simulink model "casper_sim_phase0"  (R2025b)
settings: Solver=FixedStepDiscrete  StartTime=0  StopTime=5  FixedStep=1e-3  RelTol=1e-3
undefined symbols (not defined in the file or in its folder): Estimator
libraries: imu_block_visual x2, baro_block_visual x1, gps_block_visual x1, mag_block_visual x1
settings Model: Creator=Ashwin  LastModifiedBy=Ashwin
settings DebuggingCC: InheritedTsInSrcMsg=none

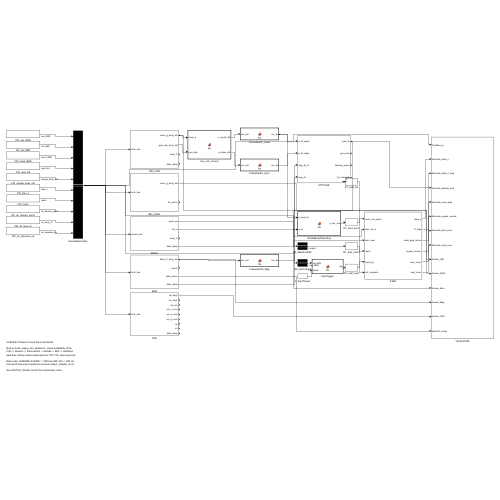
[thumbnail: Simulink's stored preview of the top-level diagram]
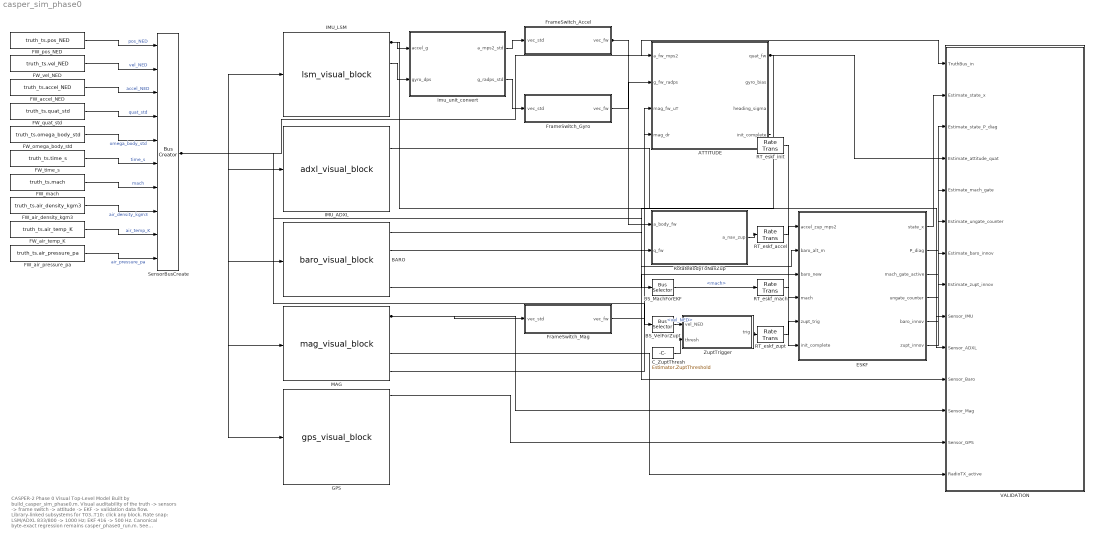
== system casper_sim_phase0 ==
  note: CASPER-2 Phase 0 Visual Top-Level Model
      |
      | Built by build_casper_sim_phase0.m. Visual auditability of the
      | truth -> sensors -> frame switch -> attitude -> EKF -> validation
      | data flow. Library-linked subsystems for T03..T10; click any block.
      |
      | Rate snap: LSM/ADXL 833/800 -> 1000 Hz; EKF 416 -> 500 Hz.
      | Canonical byte-exact regression remains casper_phase0_run.m.
      |
      | See STATUS_VISUAL.md for the construction notes.
  ATTITUDE : Subsystem
  BARO : baro_block_visual/baro_visual_block  SystemSampleTime=-1  VariantActivationTime=update diagram  EmptyChoice=off  PassThrough=off  PassThroughVariantControl=(default)  EmptyChoiceVariantControl=(default)  AllowFlexibleInterface=on  Latency=0  AutoFrameSizeCalculation=off
  BS_MachForEKF : BusSelector  OutputSignals=mach
  BS_VelForZupt : BusSelector  OutputSignals=vel_NED
  C_ZuptThresh : Constant  Value=Estimator.ZuptThreshold  SampleTime=-1
  ESKF : Subsystem
  FW_accel_NED : FromWorkspace  VariableName=truth_ts.accel_NED  SampleTime=-1  ZeroCross=off  OutputAfterFinalValue=Holding final value
  FW_air_density_kgm3 : FromWorkspace  VariableName=truth_ts.air_density_kgm3  SampleTime=-1  ZeroCross=off  OutputAfterFinalValue=Holding final value
  FW_air_pressure_pa : FromWorkspace  VariableName=truth_ts.air_pressure_pa  SampleTime=-1  ZeroCross=off  OutputAfterFinalValue=Holding final value
  FW_air_temp_K : FromWorkspace  VariableName=truth_ts.air_temp_K  SampleTime=-1  ZeroCross=off  OutputAfterFinalValue=Holding final value
  FW_mach : FromWorkspace  VariableName=truth_ts.mach  SampleTime=-1  ZeroCross=off  OutputAfterFinalValue=Holding final value
  FW_omega_body_std : FromWorkspace  VariableName=truth_ts.omega_body_std  SampleTime=-1  ZeroCross=off  OutputAfterFinalValue=Holding final value
  FW_pos_NED : FromWorkspace  VariableName=truth_ts.pos_NED  SampleTime=-1  ZeroCross=off  OutputAfterFinalValue=Holding final value
  FW_quat_std : FromWorkspace  VariableName=truth_ts.quat_std  SampleTime=-1  ZeroCross=off  OutputAfterFinalValue=Holding final value
  FW_time_s : FromWorkspace  VariableName=truth_ts.time_s  SampleTime=-1  ZeroCross=off  OutputAfterFinalValue=Holding final value
  FW_vel_NED : FromWorkspace  VariableName=truth_ts.vel_NED  SampleTime=-1  ZeroCross=off  OutputAfterFinalValue=Holding final value
  FrameSwitch_Accel : MATLAB Function  TreatAsAtomicUnit=on
  FrameSwitch_Gyro : MATLAB Function  TreatAsAtomicUnit=on
  FrameSwitch_Mag : MATLAB Function  TreatAsAtomicUnit=on
  GPS : gps_block_visual/gps_visual_block  SystemSampleTime=-1  VariantActivationTime=update diagram  EmptyChoice=off  PassThrough=off  PassThroughVariantControl=(default)  EmptyChoiceVariantControl=(default)  AllowFlexibleInterface=on  Latency=0  AutoFrameSizeCalculation=off
  IMU_ADXL : imu_block_visual/adxl_visual_block  SystemSampleTime=-1  VariantActivationTime=update diagram  EmptyChoice=off  PassThrough=off  PassThroughVariantControl=(default)  EmptyChoiceVariantControl=(default)  AllowFlexibleInterface=on  Latency=0  AutoFrameSizeCalculation=off
  IMU_LSM : imu_block_visual/lsm_visual_block  SystemSampleTime=-1  VariantActivationTime=update diagram  EmptyChoice=off  PassThrough=off  PassThroughVariantControl=(default)  EmptyChoiceVariantControl=(default)  AllowFlexibleInterface=on  Latency=0  AutoFrameSizeCalculation=off
  MAG : mag_block_visual/mag_visual_block  SystemSampleTime=-1  VariantActivationTime=update diagram  EmptyChoice=off  PassThrough=off  PassThroughVariantControl=(default)  EmptyChoiceVariantControl=(default)  AllowFlexibleInterface=on  Latency=0  AutoFrameSizeCalculation=off
  RT_eskf_accel : RateTransition  OutPortSampleTime=2e-3
  RT_eskf_init : RateTransition  OutPortSampleTime=2e-3
  RT_eskf_mach : RateTransition  OutPortSampleTime=2e-3
  RT_eskf_zupt : RateTransition  OutPortSampleTime=2e-3
  RotateBodyToNavZup : MATLAB Function  TreatAsAtomicUnit=on
  SensorBusCreate : BusCreator  Inputs=10  OutDataTypeStr=Bus: SensorInputBus  NonVirtualBus=on
  VALIDATION : Subsystem
  ZuptTrigger : MATLAB Function  TreatAsAtomicUnit=on
  imu_unit_convert : MATLAB Function  TreatAsAtomicUnit=on
  wires:
  FW_pos_NED/1 -> SensorBusCreate/1  "pos_NED"
  FW_vel_NED/1 -> SensorBusCreate/2  "vel_NED"
  FW_accel_NED/1 -> SensorBusCreate/3  "accel_NED"
  FW_quat_std/1 -> SensorBusCreate/4  "quat_std"
  FW_omega_body_std/1 -> SensorBusCreate/5  "omega_body_std"
  FW_time_s/1 -> SensorBusCreate/6  "time_s"
  FW_mach/1 -> SensorBusCreate/7  "mach"
  FW_air_density_kgm3/1 -> SensorBusCreate/8  "air_density_kgm3"
  FW_air_temp_K/1 -> SensorBusCreate/9  "air_temp_K"
  FW_air_pressure_pa/1 -> SensorBusCreate/10  "air_pressure_pa"
  SensorBusCreate/1 -> IMU_LSM/1, IMU_ADXL/1, BARO/1, MAG/1, GPS/1, BS_MachForEKF/1, BS_VelForZupt/1, VALIDATION/1(TruthBus_in)
  IMU_LSM/1 -> imu_unit_convert/1(accel_g), VALIDATION/9(Sensor_IMU)
  IMU_LSM/2 -> imu_unit_convert/2(gyro_dps)
  imu_unit_convert/1(a_mps2_std) -> FrameSwitch_Accel/1(vec_std)
  imu_unit_convert/2(g_radps_std) -> FrameSwitch_Gyro/1(vec_std)
  MAG/1 -> FrameSwitch_Mag/1(vec_std), VALIDATION/12(Sensor_Mag)
  FrameSwitch_Accel/1(vec_fw) -> ATTITUDE/1(a_fw_mps2), RotateBodyToNavZup/1(a_body_fw)
  FrameSwitch_Gyro/1(vec_fw) -> ATTITUDE/2(g_fw_radps)
  FrameSwitch_Mag/1(vec_fw) -> ATTITUDE/3(mag_fw_uT)
  MAG/4 -> ATTITUDE/4(mag_dr)
  ATTITUDE/1(quat_fw) -> RotateBodyToNavZup/2(q_fw), VALIDATION/4(Estimate_attitude_quat)
  RotateBodyToNavZup/1(a_nav_zup) -> RT_eskf_accel/1
  BS_MachForEKF/1 -> RT_eskf_mach/1  "<mach>"
  BS_VelForZupt/1 -> ZuptTrigger/1(vel_NED)  "<vel_NED>"
  C_ZuptThresh/1 -> ZuptTrigger/2(thresh)
  ZuptTrigger/1(trig) -> RT_eskf_zupt/1
  ATTITUDE/4(init_complete) -> RT_eskf_init/1
  RT_eskf_accel/1 -> ESKF/1(accel_zup_mps2)
  BARO/2 -> ESKF/2(baro_alt_m)
  BARO/4 -> ESKF/3(baro_new)
  RT_eskf_mach/1 -> ESKF/4(mach)
  RT_eskf_zupt/1 -> ESKF/5(zupt_trig)
  RT_eskf_init/1 -> ESKF/6(init_complete)
  ESKF/1(state_x) -> VALIDATION/2(Estimate_state_x)
  ESKF/2(P_diag) -> VALIDATION/3(Estimate_state_P_diag)
  ESKF/3(mach_gate_active) -> VALIDATION/5(Estimate_mach_gate)
  ESKF/4(ungate_counter) -> VALIDATION/6(Estimate_ungate_counter)
  ESKF/5(baro_innov) -> VALIDATION/7(Estimate_baro_innov)
  ESKF/6(zupt_innov) -> VALIDATION/8(Estimate_zupt_innov)
  IMU_ADXL/1 -> VALIDATION/10(Sensor_ADXL)
  BARO/1 -> VALIDATION/11(Sensor_Baro)
  GPS/1 -> VALIDATION/13(Sensor_GPS)
  MAG/3 -> VALIDATION/14(RadioTX_active)

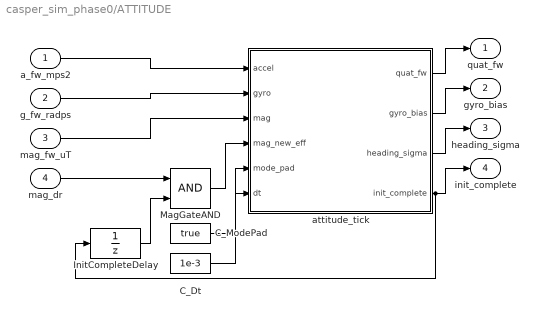
== system casper_sim_phase0/ATTITUDE ==
  a_fw_mps2 : Inport
  g_fw_radps : Inport  Port=2
  mag_fw_uT : Inport  Port=3
  mag_dr : Inport  Port=4
  C_Dt : Constant  Value=1e-3  SampleTime=-1
  C_ModePad : Constant  Value=true  OutDataTypeStr=boolean  SampleTime=-1
  InitCompleteDelay : UnitDelay  SampleTime=-1  HasFrameUpgradeWarning=on
  MagGateAND : Logic  AllPortsSameDT=off  OutDataTypeStr=boolean
  attitude_tick : MATLAB Function  TreatAsAtomicUnit=on
  quat_fw : Outport
  gyro_bias : Outport  Port=2
  heading_sigma : Outport  Port=3
  init_complete : Outport  Port=4
  wires:
  mag_dr/1 -> MagGateAND/1
  InitCompleteDelay/1 -> MagGateAND/2
  a_fw_mps2/1 -> attitude_tick/1(accel)
  g_fw_radps/1 -> attitude_tick/2(gyro)
  mag_fw_uT/1 -> attitude_tick/3(mag)
  MagGateAND/1 -> attitude_tick/4(mag_new_eff)
  C_ModePad/1 -> attitude_tick/5(mode_pad)
  C_Dt/1 -> attitude_tick/6(dt)
  attitude_tick/4(init_complete) -> InitCompleteDelay/1, init_complete/1
  attitude_tick/1(quat_fw) -> quat_fw/1
  attitude_tick/2(gyro_bias) -> gyro_bias/1
  attitude_tick/3(heading_sigma) -> heading_sigma/1

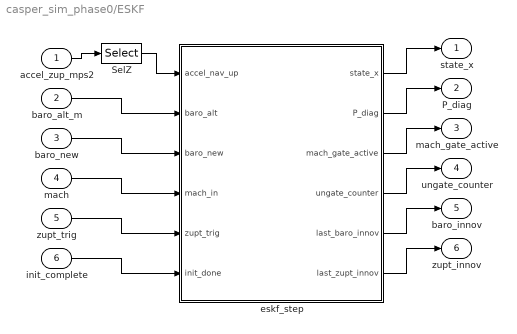
== system casper_sim_phase0/ESKF ==
  accel_zup_mps2 : Inport
  baro_alt_m : Inport  Port=2
  baro_new : Inport  Port=3
  mach : Inport  Port=4
  zupt_trig : Inport  Port=5
  init_complete : Inport  Port=6
  SelZ : Selector  InputPortWidth=3  IndexOptions=Index vector (dialog)  Indices=3  OutputSizes=1
  eskf_step : MATLAB Function  TreatAsAtomicUnit=on
  state_x : Outport
  P_diag : Outport  Port=2
  mach_gate_active : Outport  Port=3
  ungate_counter : Outport  Port=4
  baro_innov : Outport  Port=5
  zupt_innov : Outport  Port=6
  wires:
  accel_zup_mps2/1 -> SelZ/1
  SelZ/1 -> eskf_step/1(accel_nav_up)
  baro_alt_m/1 -> eskf_step/2(baro_alt)
  baro_new/1 -> eskf_step/3(baro_new)
  mach/1 -> eskf_step/4(mach_in)
  zupt_trig/1 -> eskf_step/5(zupt_trig)
  init_complete/1 -> eskf_step/6(init_done)
  eskf_step/1(state_x) -> state_x/1
  eskf_step/2(P_diag) -> P_diag/1
  eskf_step/3(mach_gate_active) -> mach_gate_active/1
  eskf_step/4(ungate_counter) -> ungate_counter/1
  eskf_step/5(last_baro_innov) -> baro_innov/1
  eskf_step/6(last_zupt_innov) -> zupt_innov/1

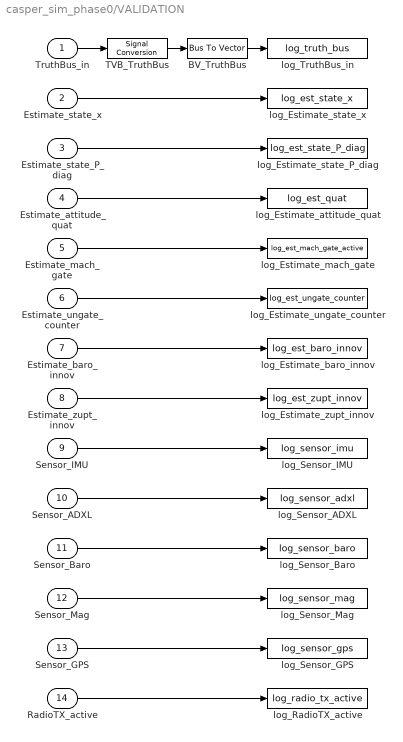
== system casper_sim_phase0/VALIDATION ==
  TruthBus_in : Inport
  Estimate_state_x : Inport  Port=2
  Estimate_state_P_diag : Inport  Port=3
  Estimate_attitude_quat : Inport  Port=4
  Estimate_mach_gate : Inport  Port=5
  Estimate_ungate_counter : Inport  Port=6
  Estimate_baro_innov : Inport  Port=7
  Estimate_zupt_innov : Inport  Port=8
  Sensor_IMU : Inport  Port=9
  Sensor_ADXL : Inport  Port=10
  Sensor_Baro : Inport  Port=11
  Sensor_Mag : Inport  Port=12
  Sensor_GPS : Inport  Port=13
  RadioTX_active : Inport  Port=14
  BV_TruthBus : BusToVector
  TVB_TruthBus : SignalConversion  ConversionOutput=Virtual bus  OverrideOpt=off
  log_Estimate_attitude_quat : ToWorkspace  VariableName=log_est_quat  SaveFormat=Structure With Time  SampleTime=-1
  log_Estimate_baro_innov : ToWorkspace  VariableName=log_est_baro_innov  SaveFormat=Structure With Time  SampleTime=-1
  log_Estimate_mach_gate : ToWorkspace  VariableName=log_est_mach_gate_active  SaveFormat=Structure With Time  SampleTime=-1
  log_Estimate_state_P_diag : ToWorkspace  VariableName=log_est_state_P_diag  SaveFormat=Structure With Time  SampleTime=-1
  log_Estimate_state_x : ToWorkspace  VariableName=log_est_state_x  SaveFormat=Structure With Time  SampleTime=-1
  log_Estimate_ungate_counter : ToWorkspace  VariableName=log_est_ungate_counter  SaveFormat=Structure With Time  SampleTime=-1
  log_Estimate_zupt_innov : ToWorkspace  VariableName=log_est_zupt_innov  SaveFormat=Structure With Time  SampleTime=-1
  log_RadioTX_active : ToWorkspace  VariableName=log_radio_tx_active  SaveFormat=Structure With Time  SampleTime=-1
  log_Sensor_ADXL : ToWorkspace  VariableName=log_sensor_adxl  SaveFormat=Structure With Time  SampleTime=-1
  log_Sensor_Baro : ToWorkspace  VariableName=log_sensor_baro  SaveFormat=Structure With Time  SampleTime=-1
  log_Sensor_GPS : ToWorkspace  VariableName=log_sensor_gps  SaveFormat=Structure With Time  SampleTime=-1
  log_Sensor_IMU : ToWorkspace  VariableName=log_sensor_imu  SaveFormat=Structure With Time  SampleTime=-1
  log_Sensor_Mag : ToWorkspace  VariableName=log_sensor_mag  SaveFormat=Structure With Time  SampleTime=-1
  log_TruthBus_in : ToWorkspace  VariableName=log_truth_bus  SaveFormat=Structure With Time  SampleTime=-1
  wires:
  TruthBus_in/1 -> TVB_TruthBus/1
  TVB_TruthBus/1 -> BV_TruthBus/1
  BV_TruthBus/1 -> log_TruthBus_in/1
  Estimate_state_x/1 -> log_Estimate_state_x/1
  Estimate_state_P_diag/1 -> log_Estimate_state_P_diag/1
  Estimate_attitude_quat/1 -> log_Estimate_attitude_quat/1
  Estimate_mach_gate/1 -> log_Estimate_mach_gate/1
  Estimate_ungate_counter/1 -> log_Estimate_ungate_counter/1
  Estimate_baro_innov/1 -> log_Estimate_baro_innov/1
  Estimate_zupt_innov/1 -> log_Estimate_zupt_innov/1
  Sensor_IMU/1 -> log_Sensor_IMU/1
  Sensor_ADXL/1 -> log_Sensor_ADXL/1
  Sensor_Baro/1 -> log_Sensor_Baro/1
  Sensor_Mag/1 -> log_Sensor_Mag/1
  Sensor_GPS/1 -> log_Sensor_GPS/1
  RadioTX_active/1 -> log_RadioTX_active/1

== matlab function casper_sim_phase0/FrameSwitch_Accel ==
  data: vec_std input; vec_fw output
function vec_fw = fcn(vec_std)
%#codegen
v = double(vec_std(:));
vec_fw = [ v(2); v(1); -v(3) ];
end

== matlab function casper_sim_phase0/imu_unit_convert ==
  data: accel_g input; a_mps2_std output; gyro_dps input; g_radps_std output
function [a_mps2_std, g_radps_std] = fcn(accel_g, gyro_dps)
%#codegen
a_mps2_std  = double(accel_g(:)) * 9.80665;
g_radps_std = double(gyro_dps(:)) * (pi/180);
end

== matlab function casper_sim_phase0/FrameSwitch_Gyro ==
  data: vec_std input; vec_fw output
function vec_fw = fcn(vec_std)
%#codegen
v = double(vec_std(:));
vec_fw = [ v(2); v(1); -v(3) ];
end

== matlab function casper_sim_phase0/FrameSwitch_Mag ==
  data: vec_std input; vec_fw output
function vec_fw = fcn(vec_std)
%#codegen
v = double(vec_std(:));
vec_fw = [ v(2); v(1); -v(3) ];
end

== matlab function casper_sim_phase0/ATTITUDE/attitude_tick ==
  data: accel input; quat_fw output; gyro input; mag input; mag_new_eff input; mode_pad input; dt input; gyro_bias output; heading_sigma output; init_complete output
function [quat_fw, gyro_bias, heading_sigma, init_complete] = fcn(accel, gyro, mag, mag_new_eff, mode_pad, dt)
%#codegen
coder.extrinsic('attitude_step_helper');
% Preallocate outputs so chart parser can infer types.
quat_fw       = [1;0;0;0];
gyro_bias     = zeros(3,1);
heading_sigma = double(0);
init_complete = false;
[quat_fw, gyro_bias, heading_sigma, init_complete] = attitude_step_helper(double(accel), double(gyro), double(mag), logical(mag_new_eff), logical(mode_pad), double(dt));
end

== matlab function casper_sim_phase0/ESKF/eskf_step ==
  data: accel_nav_up input; state_x output; baro_alt input; baro_new input; mach_in input; zupt_trig input; init_done input; P_diag output; mach_gate_active output; ungate_counter output; last_baro_innov output; last_zupt_innov output
function [state_x, P_diag, mach_gate_active, ungate_counter, last_baro_innov, last_zupt_innov] = fcn(accel_nav_up, baro_alt, baro_new, mach_in, zupt_trig, init_done)
%#codegen
coder.extrinsic('eskf_step_helper');
% All outputs preallocated to fixed sizes so the chart parser can
% statically infer types even with extrinsic call.
state_x = zeros(4,1);
P_diag  = zeros(4,1);
mach_gate_active = double(0);
ungate_counter   = double(0);
last_baro_innov  = double(0);
last_zupt_innov  = double(0);
[state_x, P_diag, mach_gate_active, ungate_counter, last_baro_innov, last_zupt_innov] = eskf_step_helper(double(accel_nav_up), double(baro_alt), logical(baro_new), double(mach_in), logical(zupt_trig), logical(init_done));
end

== matlab function casper_sim_phase0/RotateBodyToNavZup ==
  data: a_body_fw input; a_nav_zup output; q_fw input
function a_nav_zup = fcn(a_body_fw, q_fw)
%#codegen
q = double(q_fw(:));
a = double(a_body_fw(:));
nq = sqrt(q(1)*q(1)+q(2)*q(2)+q(3)*q(3)+q(4)*q(4));
if nq < 1e-12; nq = 1; end
q = q / nq;
w = q(1); x = q(2); y = q(3); z = q(4);
R = [1-2*(y*y+z*z),   2*(x*y - z*w),   2*(x*z + y*w);
     2*(x*y + z*w),   1-2*(x*x+z*z),   2*(y*z - x*w);
     2*(x*z - y*w),   2*(y*z + x*w),   1-2*(x*x+y*y)];
a_nav_zup = R * a;
end

== matlab function casper_sim_phase0/ZuptTrigger ==
  data: vel_NED input; trig output; thresh input
function trig = fcn(vel_NED, thresh)
%#codegen
v = double(vel_NED(:));
trig = sqrt(v(1)^2 + v(2)^2 + v(3)^2) < double(thresh);
end
